simulink model "Quad_Nonlinear_Pitch_Model"  (R2020a)
settings: Solver=ode3  StartTime=0.0  StopTime=20  FixedStep=0.02  RelTol=1e-3  EnableMultiTasking=on
InitFcn:
  | LQR_Solver;
undefined symbols (not defined in the file or in its folder): B1, B5, Ba, K
libraries: simulink x2, eeGeneralControl x2, pil_lib x1
settings Model: SILPILModeSetting=veronly  ExtModeTrigDuration=2  Creator=Ali  LastModifiedBy=Ali
settings OptimizationCC: DefaultUnderspecifiedDataType=single  EnhancedBackFolding=on  PassReuseOutputArgsAs=Individual arguments  ZeroExternalMemoryAtStartup=off  ZeroInternalMemoryAtStartup=off  MaxStackSize=64  OptimizeBlockOrder=speed  DifferentSizesBufferReuse=on  OptimizationCustomize=off  EfficientTunableParamExpr=on
settings DebuggingCC: ParameterPrecisionLossMsg=none  ParameterTunabilityLossMsg=error
settings HardwareCC: ProdBitPerInt=16  ProdBitPerPointer=16  ProdBitPerSizeT=16  ProdBitPerPtrDiffT=16  ProdLargestAtomicFloat=None  ProdWordSize=8  ProdHWDeviceType=Atmel->AVR
settings SFSimCC: MATLABDynamicMemAlloc=off
settings RTWCC: SystemTargetFile=ert.tlc  HardwareBoard=Arduino Mega 2560  TLCOptions=-aInlineSetEventsForThisBaseRateFcn=TLC_FALSE -aSuppressMultiTaskScheduler=TLC_FALSE -aRateBasedStepFcn=1  TemplateMakefile=ert_default_tmf  Toolchain=Arduino AVR  BuildConfiguration=Faster Runs  CreateSILPILBlock=PIL
settings CodeAppCC: ForceParamTrailComments=on  IgnoreCustomStorageClasses=off  OperatorAnnotations=on  SimulinkDataObjDesc=on  SFDataObjDesc=on  InsertBlockDesc=on
settings ERTTargetCC: TargetLangStandard=C99 (ISO)  SupportContinuousTime=on  SupportVariableSizeSignals=on  ExtModeStaticAllocSize=2048

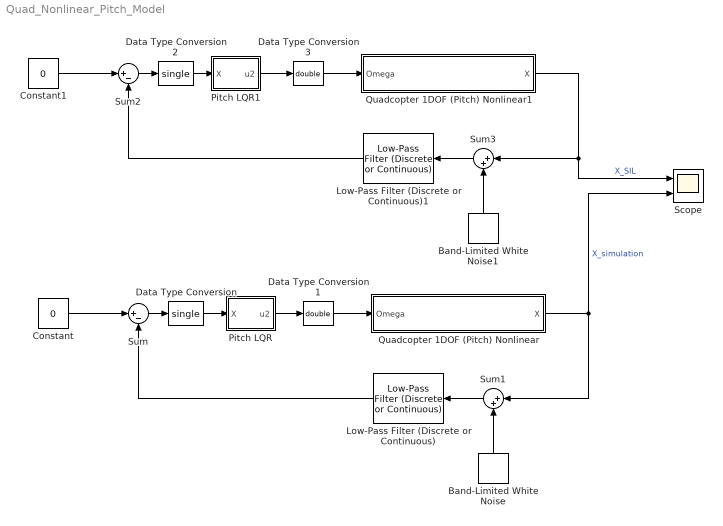
== system Quad_Nonlinear_Pitch_Model ==
  Band-Limited White Noise : simulink/Sources/Band-Limited White Noise  Cov=[0.0001]  Ts=0.02  seed=[23341]
  Band-Limited White Noise1 : simulink/Sources/Band-Limited White Noise  Cov=[0.0001]  Ts=0.02  seed=[23341]
  Constant : Constant  Value=0
  Constant1 : Constant  Value=0
  Data Type Conversion : DataTypeConversion  OutDataTypeStr=single
  Data Type Conversion1 : DataTypeConversion  OutDataTypeStr=double
  Data Type Conversion2 : DataTypeConversion  OutDataTypeStr=single
  Data Type Conversion3 : DataTypeConversion  OutDataTypeStr=double
  Low-Pass Filter (Discrete or Continuous) : eeGeneralControl/Low-Pass Filter (Discrete or Continuous)  K=1  T=0.05  B=inf  A=-inf  init_option=Inherited from block input  x0=0  Ts=0
  Low-Pass Filter (Discrete or Continuous)1 : eeGeneralControl/Low-Pass Filter (Discrete or Continuous)  K=1  T=0.05  B=inf  A=-inf  init_option=Inherited from block input  x0=0  Ts=0
  Pitch LQR : Subsystem
  Pitch LQR1 : Subsystem  DialogController=pil_create_dialog  LoadFcn=|
      | try
      |    if ~strcmp(rtw.pil.getPILVersion, '9.8 (R2020a)_13')
      |       set_param(gcb, 'DialogController', '');
      |       set_param(gcb, 'DialogControllerArgs', '');
      |    end
      | catch e
      |       set_param(gcb, 'DialogController', '');
      |       set_param(gcb, 'DialogControllerArgs', '');
      | end
      mask help: PIL:pil:XILBlockMaskDesc
      mask Display: disp('SIL');
  Quadcopter 1DOF (Pitch) Nonlinear : Subsystem  TreatAsAtomicUnit=on
      mask Display: image('Seesaw.png'); % Use "Edit Image" on toolstrip to change.
  Quadcopter 1DOF (Pitch) Nonlinear1 : Subsystem  TreatAsAtomicUnit=on
      mask Display: image('Seesaw.png'); % Use "Edit Image" on toolstrip to change.
  Scope : Scope  NumInputPorts=2
  Sum : Sum  Inputs=|+-
  Sum1 : Sum  Inputs=|++
  Sum2 : Sum  Inputs=|+-
  Sum3 : Sum  Inputs=|++
  wires:
  Quadcopter 1DOF (Pitch) Nonlinear/1(X) -> Scope/2, Sum1/1  "X_simulation"
  Constant/1 -> Sum/1
  Band-Limited White Noise/1 -> Sum1/2
  Sum1/1 -> Low-Pass Filter (Discrete or Continuous)/1
  Pitch LQR/1(u2) -> Data Type Conversion1/1
  Low-Pass Filter (Discrete or Continuous)/1 -> Sum/2
  Sum/1 -> Data Type Conversion/1
  Data Type Conversion1/1 -> Quadcopter 1DOF (Pitch) Nonlinear/1(Omega)
  Data Type Conversion/1 -> Pitch LQR/1(X)
  Constant1/1 -> Sum2/1
  Sum2/1 -> Data Type Conversion2/1
  Quadcopter 1DOF (Pitch) Nonlinear1/1(X) -> Scope/1, Sum3/1  "X_SIL"
  Sum3/1 -> Low-Pass Filter (Discrete or Continuous)1/1
  Low-Pass Filter (Discrete or Continuous)1/1 -> Sum2/2
  Band-Limited White Noise1/1 -> Sum3/2
  Pitch LQR1/1(u2) -> Data Type Conversion3/1
  Data Type Conversion3/1 -> Quadcopter 1DOF (Pitch) Nonlinear1/1(Omega)
  Data Type Conversion2/1 -> Pitch LQR1/1(X)

== system Quad_Nonlinear_Pitch_Model/Pitch LQR ==
  X : Inport
  Constant : Constant  Value=K  OutDataTypeStr=Inherit: Inherit via back propagation
  Product : Product  Multiplication=Matrix(*)
  u2 : Outport
  wires:
  Product/1 -> u2/1
  Constant/1 -> Product/2
  X/1 -> Product/1

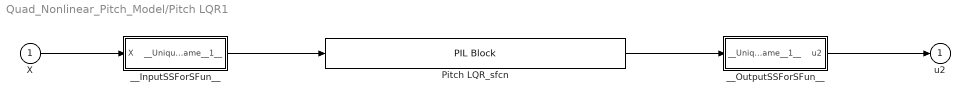
== system Quad_Nonlinear_Pitch_Model/Pitch LQR1 ==
  X : Inport
  Pitch LQR_sfcn : pil_lib/PIL Block  SimulationMode=SIL  IsTopModelPIL=off  CodeDir=/Users/Ali/Documents/BAI/Aerospace/bachelor-thesis/Code/Simulink/Quadcopter/SIL/LQR/Pitch/Pitch_ert_rtw  AnchorDir=/Users/Ali/Documents/BAI/Aerospace/bachelor-thesis/Code/Simulink/Quadcopter/SIL/LQR/Pitch  ConfigName=Software-in-the-Loop (SIL)  XrelIsTopModelCode=on  XrelIsReusable=off  XrelDWorkNames={}  XrelDWorkTypes={}  XrelModelArgVals={}  XrelOrderedParamNames={}
      settings: SourceProductBaseCode=RT
  __InputSSForSFun__ : Subsystem
  __OutputSSForSFun__ : Subsystem
  u2 : Outport
  wires:
  X/1 -> __InputSSForSFun__/1(X)
  __InputSSForSFun__/1(__UniqueOutportName__1__) -> Pitch LQR_sfcn/1
  Pitch LQR_sfcn/1 -> __OutputSSForSFun__/1(__UniqueInportName__1__)
  __OutputSSForSFun__/1(u2) -> u2/1

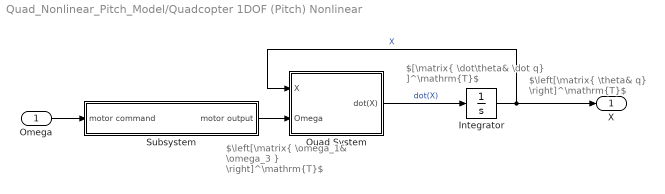
== system Quad_Nonlinear_Pitch_Model/Quadcopter 1DOF (Pitch) Nonlinear ==
  note: $\left[\matrix{ \omega_1& \omega_3 } \right]^\mathrm{T}$
  note: $\left[\matrix{ \theta& q} \right]^\mathrm{T}$
  note: $[\matrix{ \dot\theta& \dot q} ]^\mathrm{T}$
  Omega : Inport
  Integrator : Integrator  InitialCondition=[0.9628, 0]
  Quad System : Subsystem
  Subsystem : Subsystem
  X : Outport
  wires:
  Integrator/1 -> X/1, Quad System/1(X)  "X"
  Quad System/1(dot(X)) -> Integrator/1  "dot(X)"
  Omega/1 -> Subsystem/1(motor command)
  Subsystem/1(motor output) -> Quad System/2(Omega)

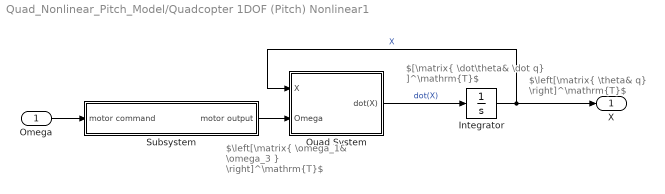
== system Quad_Nonlinear_Pitch_Model/Quadcopter 1DOF (Pitch) Nonlinear1 ==
  note: $\left[\matrix{ \omega_1& \omega_3 } \right]^\mathrm{T}$
  note: $\left[\matrix{ \theta& q} \right]^\mathrm{T}$
  note: $[\matrix{ \dot\theta& \dot q} ]^\mathrm{T}$
  Omega : Inport
  Integrator : Integrator  InitialCondition=[0.9628, 0]
  Quad System : Subsystem
  Subsystem : Subsystem
  X : Outport
  wires:
  Integrator/1 -> X/1, Quad System/1(X)  "X"
  Quad System/1(dot(X)) -> Integrator/1  "dot(X)"
  Omega/1 -> Subsystem/1(motor command)
  Subsystem/1(motor output) -> Quad System/2(Omega)

== system Quad_Nonlinear_Pitch_Model/Pitch LQR1/__InputSSForSFun__ ==
  X : Inport
  __UniqueOutportName__1__ : Outport
  wires:
  X/1 -> __UniqueOutportName__1__/1

== system Quad_Nonlinear_Pitch_Model/Pitch LQR1/__OutputSSForSFun__ ==
  __UniqueInportName__1__ : Inport
  u2 : Outport
  wires:
  __UniqueInportName__1__/1 -> u2/1

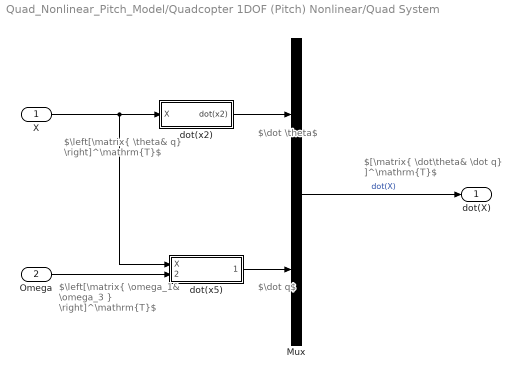
== system Quad_Nonlinear_Pitch_Model/Quadcopter 1DOF (Pitch) Nonlinear/Quad System ==
  note: $\dot \theta$
  note: $\left[\matrix{ \theta& q} \right]^\mathrm{T}$
  note: $[\matrix{ \dot\theta& \dot q} ]^\mathrm{T}$
  note: $\left[\matrix{ \omega_1& \omega_3 } \right]^\mathrm{T}$
  note: $\dot q$
  X : Inport
  Omega : Inport  Port=2
  Mux : Mux  Inputs=2
  dot(x2) : Subsystem
  dot(x5) : Subsystem
  dot(X) : Outport
  wires:
  Mux/1 -> dot(X)/1  "dot(X)"
  dot(x2)/1(dot(x2)) -> Mux/1
  dot(x5)/1(dot(x5)) -> Mux/2
  X/1 -> dot(x5)/1(X), dot(x2)/1(X)
  Omega/1 -> dot(x5)/2(Omega)

== system Quad_Nonlinear_Pitch_Model/Quadcopter 1DOF (Pitch) Nonlinear/Subsystem ==
  motor command : Inport
  Delay : Delay  DelayLength=1
  Transfer Fcn : TransferFcn  Denominator=[0.15 1]
  motor output : Outport
  wires:
  Transfer Fcn/1 -> motor output/1
  motor command/1 -> Delay/1
  Delay/1 -> Transfer Fcn/1

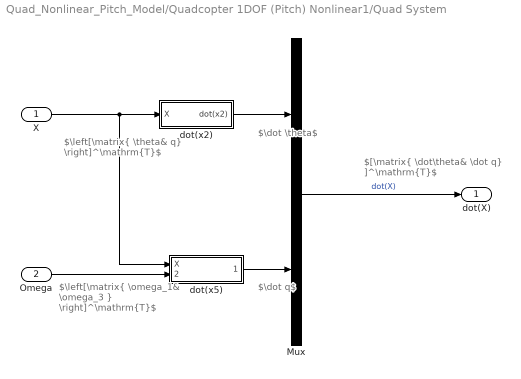
== system Quad_Nonlinear_Pitch_Model/Quadcopter 1DOF (Pitch) Nonlinear1/Quad System ==
  note: $\dot \theta$
  note: $\left[\matrix{ \theta& q} \right]^\mathrm{T}$
  note: $[\matrix{ \dot\theta& \dot q} ]^\mathrm{T}$
  note: $\left[\matrix{ \omega_1& \omega_3 } \right]^\mathrm{T}$
  note: $\dot q$
  X : Inport
  Omega : Inport  Port=2
  Mux : Mux  Inputs=2
  dot(x2) : Subsystem
  dot(x5) : Subsystem
  dot(X) : Outport
  wires:
  Mux/1 -> dot(X)/1  "dot(X)"
  dot(x2)/1(dot(x2)) -> Mux/1
  dot(x5)/1(dot(x5)) -> Mux/2
  X/1 -> dot(x5)/1(X), dot(x2)/1(X)
  Omega/1 -> dot(x5)/2(Omega)

== system Quad_Nonlinear_Pitch_Model/Quadcopter 1DOF (Pitch) Nonlinear1/Subsystem ==
  motor command : Inport
  Delay : Delay  DelayLength=1
  Transfer Fcn : TransferFcn  Denominator=[0.15 1]
  motor output : Outport
  wires:
  Transfer Fcn/1 -> motor output/1
  motor command/1 -> Delay/1
  Delay/1 -> Transfer Fcn/1

== system Quad_Nonlinear_Pitch_Model/Quadcopter 1DOF (Pitch) Nonlinear/Quad System/dot(x2) ==
  X : Inport
  1 : Subsystem
  dot(x2) : Outport
  wires:
  X/1 -> 1/1(X)  "X"
  1/1(x5cos(x1)) -> dot(x2)/1

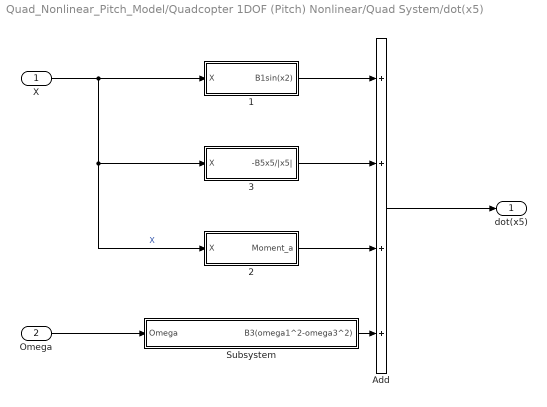
== system Quad_Nonlinear_Pitch_Model/Quadcopter 1DOF (Pitch) Nonlinear/Quad System/dot(x5) ==
  X : Inport
  Omega : Inport  Port=2
  1 : Subsystem
  2 : Subsystem
  3 : Subsystem
  Add : Sum  Inputs=++++
  Subsystem : Subsystem
  dot(x5) : Outport
  wires:
  X/1 -> 2/1(X), 3/1(X), 1/1(X)  "X"
  Omega/1 -> Subsystem/1(Omega)
  Add/1 -> dot(x5)/1
  3/1("-B5x5/|x5| ") -> Add/2
  1/1(B1sin(x2)) -> Add/1
  Subsystem/1(B3(omega1^2-omega3^2)) -> Add/4
  2/1(Moment_a) -> Add/3

== system Quad_Nonlinear_Pitch_Model/Quadcopter 1DOF (Pitch) Nonlinear1/Quad System/dot(x2) ==
  X : Inport
  1 : Subsystem
  dot(x2) : Outport
  wires:
  X/1 -> 1/1(X)  "X"
  1/1(x5cos(x1)) -> dot(x2)/1

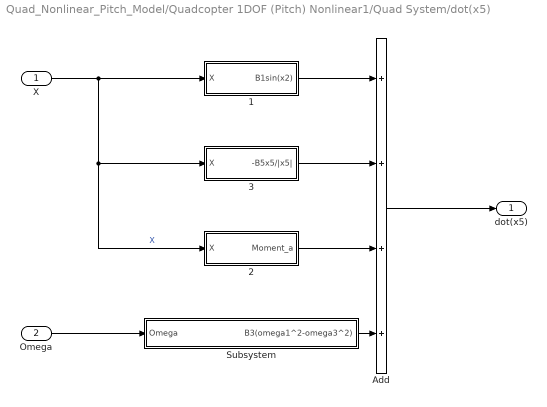
== system Quad_Nonlinear_Pitch_Model/Quadcopter 1DOF (Pitch) Nonlinear1/Quad System/dot(x5) ==
  X : Inport
  Omega : Inport  Port=2
  1 : Subsystem
  2 : Subsystem
  3 : Subsystem
  Add : Sum  Inputs=++++
  Subsystem : Subsystem
  dot(x5) : Outport
  wires:
  X/1 -> 2/1(X), 3/1(X), 1/1(X)  "X"
  Omega/1 -> Subsystem/1(Omega)
  Add/1 -> dot(x5)/1
  3/1("-B5x5/|x5| ") -> Add/2
  1/1(B1sin(x2)) -> Add/1
  Subsystem/1(B3(omega1^2-omega3^2)) -> Add/4
  2/1(Moment_a) -> Add/3

== system Quad_Nonlinear_Pitch_Model/Quadcopter 1DOF (Pitch) Nonlinear/Quad System/dot(x2)/1 ==
  X : Inport
  Selector : Selector  InputPortWidth=2  IndexOptions=Index vector (dialog)  Indices=[2]  OutputSizes=1
  x5cos(x1) : Outport
  wires:
  X/1 -> Selector/1  "x"
  Selector/1 -> x5cos(x1)/1

== system Quad_Nonlinear_Pitch_Model/Quadcopter 1DOF (Pitch) Nonlinear/Quad System/dot(x5)/1 ==
  X : Inport
  Selector : Selector  InputPortWidth=2  IndexOptions=Index vector (dialog)  Indices=[1]  OutputSizes=1
  Subsystem : Subsystem
  B1sin(x2) : Outport
  wires:
  X/1 -> Selector/1  "x"
  Subsystem/1(B1sin(x2)) -> B1sin(x2)/1
  Selector/1 -> Subsystem/1(x2)

== system Quad_Nonlinear_Pitch_Model/Quadcopter 1DOF (Pitch) Nonlinear/Quad System/dot(x5)/2 ==
  X : Inport
  Selector : Selector  InputPortWidth=2  IndexOptions=Index vector (dialog)  Indices=[1]  OutputSizes=1
  Subsystem : Subsystem
  Moment_a : Outport
  wires:
  X/1 -> Selector/1  "x"
  Subsystem/1(moment_a) -> Moment_a/1
  Selector/1 -> Subsystem/1(In1)

== system Quad_Nonlinear_Pitch_Model/Quadcopter 1DOF (Pitch) Nonlinear/Quad System/dot(x5)/3 ==
  X : Inport
  Selector : Selector  InputPortWidth=2  IndexOptions=Index vector (dialog)  Indices=[2]  OutputSizes=1
  Subsystem : Subsystem
  "-B5x5/|x5| " : Outport
  wires:
  X/1 -> Selector/1  "x"
  Subsystem/1("-B5x5/|x5| ") -> "-B5x5/|x5| "/1
  Selector/1 -> Subsystem/1(x5)

== system Quad_Nonlinear_Pitch_Model/Quadcopter 1DOF (Pitch) Nonlinear/Quad System/dot(x5)/Subsystem ==
  Omega : Inport
  B3(omega1^2-omega3^2) : Outport
  wires:
  Omega/1 -> B3(omega1^2-omega3^2)/1

== system Quad_Nonlinear_Pitch_Model/Quadcopter 1DOF (Pitch) Nonlinear1/Quad System/dot(x2)/1 ==
  X : Inport
  Selector : Selector  InputPortWidth=2  IndexOptions=Index vector (dialog)  Indices=[2]  OutputSizes=1
  x5cos(x1) : Outport
  wires:
  X/1 -> Selector/1  "x"
  Selector/1 -> x5cos(x1)/1

== system Quad_Nonlinear_Pitch_Model/Quadcopter 1DOF (Pitch) Nonlinear1/Quad System/dot(x5)/1 ==
  X : Inport
  Selector : Selector  InputPortWidth=2  IndexOptions=Index vector (dialog)  Indices=[1]  OutputSizes=1
  Subsystem : Subsystem
  B1sin(x2) : Outport
  wires:
  X/1 -> Selector/1  "x"
  Subsystem/1(B1sin(x2)) -> B1sin(x2)/1
  Selector/1 -> Subsystem/1(x2)

== system Quad_Nonlinear_Pitch_Model/Quadcopter 1DOF (Pitch) Nonlinear1/Quad System/dot(x5)/2 ==
  X : Inport
  Selector : Selector  InputPortWidth=2  IndexOptions=Index vector (dialog)  Indices=[1]  OutputSizes=1
  Subsystem : Subsystem
  Moment_a : Outport
  wires:
  X/1 -> Selector/1  "x"
  Subsystem/1(moment_a) -> Moment_a/1
  Selector/1 -> Subsystem/1(In1)

== system Quad_Nonlinear_Pitch_Model/Quadcopter 1DOF (Pitch) Nonlinear1/Quad System/dot(x5)/3 ==
  X : Inport
  Selector : Selector  InputPortWidth=2  IndexOptions=Index vector (dialog)  Indices=[2]  OutputSizes=1
  Subsystem : Subsystem
  "-B5x5/|x5| " : Outport
  wires:
  X/1 -> Selector/1  "x"
  Subsystem/1("-B5x5/|x5| ") -> "-B5x5/|x5| "/1
  Selector/1 -> Subsystem/1(x5)

== system Quad_Nonlinear_Pitch_Model/Quadcopter 1DOF (Pitch) Nonlinear1/Quad System/dot(x5)/Subsystem ==
  Omega : Inport
  B3(omega1^2-omega3^2) : Outport
  wires:
  Omega/1 -> B3(omega1^2-omega3^2)/1

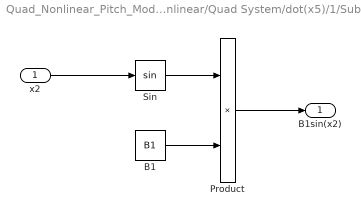
== system Quad_Nonlinear_Pitch_Model/Quadcopter 1DOF (Pitch) Nonlinear/Quad System/dot(x5)/1/Subsystem ==
  x2 : Inport
  B1 : Constant  Value=B1
  Product : Product
  Sin : Trigonometry
  B1sin(x2) : Outport
  wires:
  Product/1 -> B1sin(x2)/1
  x2/1 -> Sin/1
  B1/1 -> Product/2
  Sin/1 -> Product/1

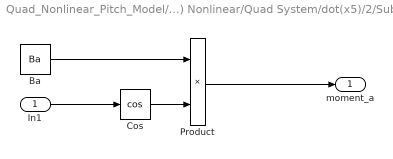
== system Quad_Nonlinear_Pitch_Model/Quadcopter 1DOF (Pitch) Nonlinear/Quad System/dot(x5)/2/Subsystem ==
  In1 : Inport
  Ba : Constant  Value=Ba
  Cos : Trigonometry  Operator=cos
  Product : Product
  moment_a : Outport
  wires:
  Product/1 -> moment_a/1
  Ba/1 -> Product/1
  In1/1 -> Cos/1
  Cos/1 -> Product/2

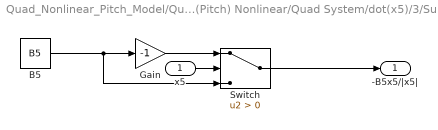
== system Quad_Nonlinear_Pitch_Model/Quadcopter 1DOF (Pitch) Nonlinear/Quad System/dot(x5)/3/Subsystem ==
  x5 : Inport
  B5 : Constant  Value=B5
  Gain : Gain  Gain=-1
  Switch : Switch  Criteria=u2 > Threshold
  "-B5x5/|x5| " : Outport
  wires:
  Switch/1 -> "-B5x5/|x5| "/1
  B5/1 -> Switch/3, Gain/1
  x5/1 -> Switch/2
  Gain/1 -> Switch/1

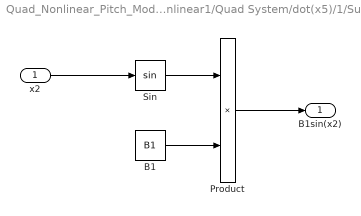
== system Quad_Nonlinear_Pitch_Model/Quadcopter 1DOF (Pitch) Nonlinear1/Quad System/dot(x5)/1/Subsystem ==
  x2 : Inport
  B1 : Constant  Value=B1
  Product : Product
  Sin : Trigonometry
  B1sin(x2) : Outport
  wires:
  Product/1 -> B1sin(x2)/1
  x2/1 -> Sin/1
  B1/1 -> Product/2
  Sin/1 -> Product/1

== system Quad_Nonlinear_Pitch_Model/Quadcopter 1DOF (Pitch) Nonlinear1/Quad System/dot(x5)/2/Subsystem ==
  In1 : Inport
  Ba : Constant  Value=Ba
  Cos : Trigonometry  Operator=cos
  Product : Product
  moment_a : Outport
  wires:
  Product/1 -> moment_a/1
  Ba/1 -> Product/1
  In1/1 -> Cos/1
  Cos/1 -> Product/2

== system Quad_Nonlinear_Pitch_Model/Quadcopter 1DOF (Pitch) Nonlinear1/Quad System/dot(x5)/3/Subsystem ==
  x5 : Inport
  B5 : Constant  Value=B5
  Gain : Gain  Gain=-1
  Switch : Switch  Criteria=u2 > Threshold
  "-B5x5/|x5| " : Outport
  wires:
  Switch/1 -> "-B5x5/|x5| "/1
  B5/1 -> Switch/3, Gain/1
  x5/1 -> Switch/2
  Gain/1 -> Switch/1
